simulink model "Model_RunAll"  (R2021b)
settings: Solver=FixedStepDiscrete  StartTime=0.0  StopTime=m.sys.tsim  FixedStep=p.sys.samp.tsim
values from neighbouring files (symbols this model uses):
  m = ConvertToDoublePrecision(m)    [Params.m]
  pp = Simulink.Parameter(p_single)    [Params.m]
settings Model: Creator=hamid.behjati  LastModifiedBy=behjati
settings DebuggingCC: AlgebraicLoopMsg=none  ParameterPrecisionLossMsg=none

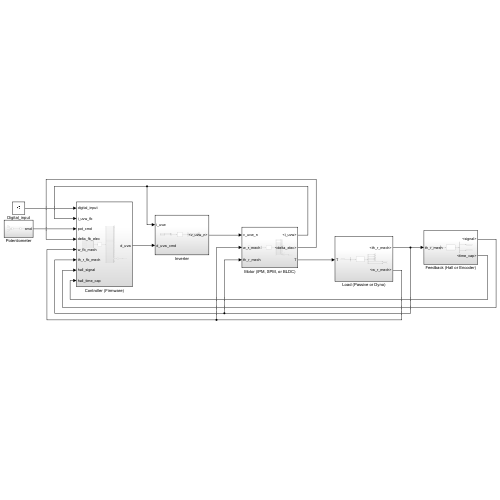
[thumbnail: Simulink's stored preview of the top-level diagram]
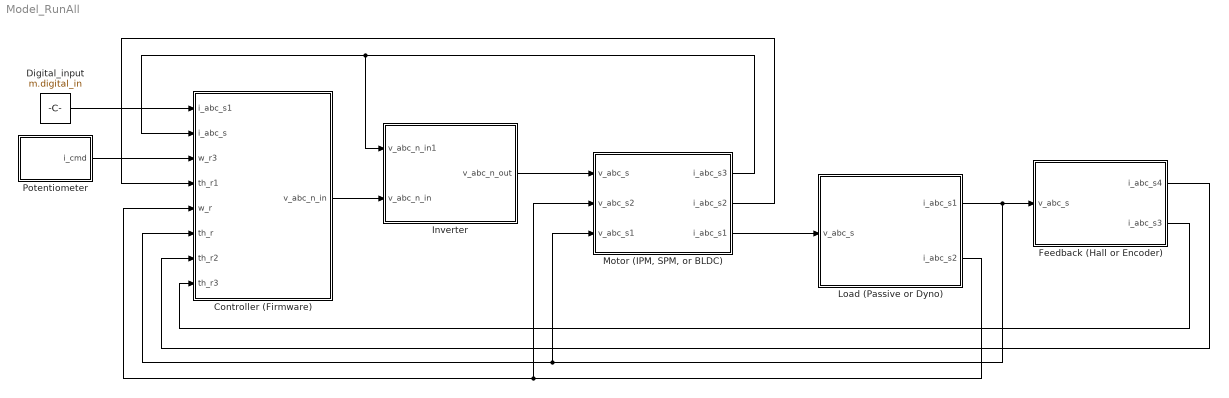
== system Model_RunAll ==
  Controller (Firmware) : Subsystem
  Digital_input : Constant  Value=m.digital_in
  Feedback (Hall or Encoder) : Subsystem
  Inverter : Subsystem
  Load (Passive or Dyno) : Subsystem
  "Motor (IPM, SPM, or BLDC)" : Subsystem
  Potentiometer : Subsystem
  wires:
  "Motor (IPM, SPM, or BLDC)"/3(i_abc_s1) -> Load (Passive or Dyno)/1(v_abc_s)
  "Motor (IPM, SPM, or BLDC)"/1(i_abc_s3) -> Controller (Firmware)/2(i_abc_s), Inverter/1(v_abc_n_in1)
  Potentiometer/1(i_cmd) -> Controller (Firmware)/3(w_r3)
  Controller (Firmware)/1(v_abc_n_in) -> Inverter/2(v_abc_n_in)
  Inverter/1(v_abc_n_out) -> "Motor (IPM, SPM, or BLDC)"/1(v_abc_s)
  Load (Passive or Dyno)/1(i_abc_s1) -> Feedback (Hall or Encoder)/1(v_abc_s), "Motor (IPM, SPM, or BLDC)"/3(v_abc_s1), Controller (Firmware)/6(th_r)
  "Motor (IPM, SPM, or BLDC)"/2(i_abc_s2) -> Controller (Firmware)/4(th_r1)
  Digital_input/1 -> Controller (Firmware)/1(i_abc_s1)
  Load (Passive or Dyno)/2(i_abc_s2) -> "Motor (IPM, SPM, or BLDC)"/2(v_abc_s2), Controller (Firmware)/5(w_r)
  Feedback (Hall or Encoder)/2(i_abc_s3) -> Controller (Firmware)/8(th_r3)
  Feedback (Hall or Encoder)/1(i_abc_s4) -> Controller (Firmware)/7(th_r2)

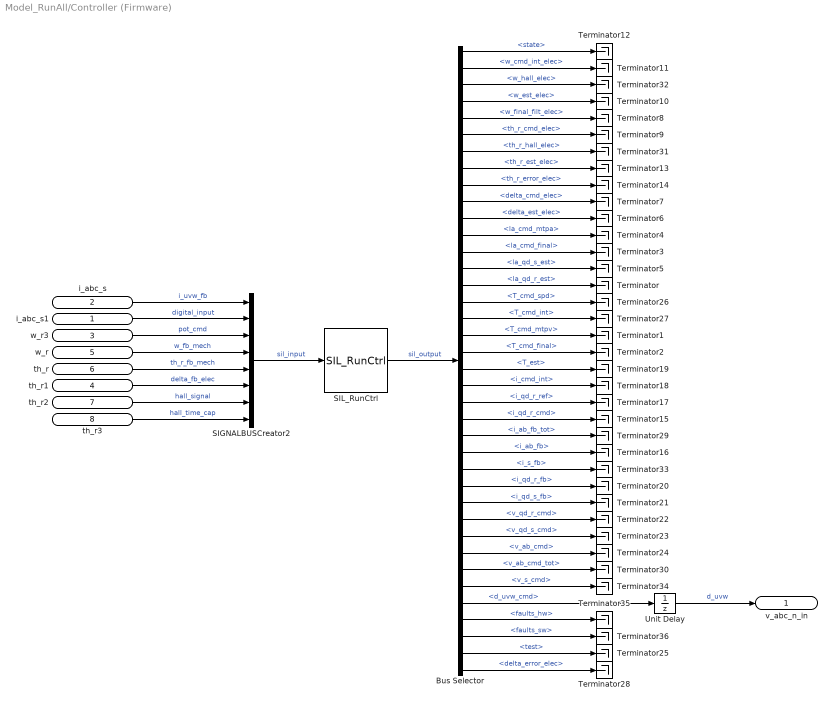
== system Model_RunAll/Controller (Firmware) ==
  i_abc_s1 : Inport
  i_abc_s : Inport  Port=2
  w_r3 : Inport  Port=3
  th_r1 : Inport  Port=4
  w_r : Inport  Port=5
  th_r : Inport  Port=6
  th_r2 : Inport  Port=7
  th_r3 : Inport  Port=8
  Bus Selector : BusSelector  OutputSignals=state,w_cmd_int_elec,w_hall_elec,w_est_elec,w_final_filt_elec,th_r_cmd_elec,th_r_hall_elec,th_r_est_elec,th_r_error_elec,delta_cmd_elec,delta_est_elec,la_cmd_mtpa,la_cmd_final,la_qd_s_est,la_qd_r_est,T_cmd_spd,T_cmd_int,T_cmd_mtpv,T_cmd_final,T_est,i_cmd_int,i_qd_r_ref,i_qd_r_cmd,i_ab_fb_tot,i_ab_fb,i_s_fb,i_qd_r_fb,i_qd_s_fb,v_qd_r_cmd,v_qd_s_cmd,v_ab_cmd,v_ab_cmd_tot,v_s_cmd,d_uvw_cmd,faults_hw,faults_sw,test,delta_error_elec
  SIGNALBUSCreator2 : BusCreator  Inputs=8  OutDataTypeStr=Bus: SIL_INPUT_CTRL_t
      settings: InheritFromInputs=off
  SIL_RunCtrl : S-Function  FunctionName=SIL_RunCtrl  Parameters=SParameter1  SFunctionDeploymentMode=off  EnableBusSupport=off  mask(Legacy Function){SFunctionSpec=void SIL_RunCtrl(SIL_INPUT_CTRL_t u1[1], SIL_OUTPUT_CTRL_t y1[1]), SParameter1=pp, ShowSpec=off}
      mask prompts: SParameter1 "P1:"; ShowSpec "Display function specification"
      mask help:
      | This block allows you to call the legacy functions specified by the following Legacy Code Tool definition:
      | def.SFunctionName = 'SIL_RunCtrl';
      | def.OutputFcnSpec = 'void SIL_RunCtrl(SIL_INPUT_CTRL_t u1[1], SIL_OUTPUT_CTRL_t y1[1])';
      | def.StartFcnSpec = 'void SIL_StartCtrl(PARAMS_t p1[1])';
      | def.TerminateFcnSpec = 'void SIL_TerminateCtrl()';
      | def.HeaderFiles = {'SILWrap.h'};
      | def.SourceFiles = {'Biquad.c', 'Controller.c', 'CtrlFilts.c', 'CtrlVars.c', 'FaultProtect.c', 'FluxWeaken.c', 'General.c', 'Observer.c', 'Params.c', 'PLL.c', 'ResonantFilt.c', 'SensorIface.c', 'SixPulseInj.c', 'SpeedCtrl.c', 'StateMachine.c', 'VoltCtrl.c', 'VoltMod.c', 'CInverter.cpp', 'CMechLoad.cpp', 'CMotor.cpp', 'AuxMethods.cpp', 'CPotentiometer.cpp', 'SILAuxFcns.cpp', 'SILWrap.cpp', 'DeltaCtrl.c', 'FluxCtrl.c', 'TrqCtrl.c'};
      | def.IncPaths = {'..\UnitTests\', '..\OperationalCode\'};
      | def.SrcPaths = {'..\UnitTests\', '..\OperationalCode\'};
      | def.SampleTime = 9.99999974737875e-06;
      mask Help: <p>This block was generated automatically by the Legacy Code Tool. For detailed help on this tool, call<a href="matlab:legacy_code('help')"> legacy_code('help')</a>.</p>
      mask Callback ShowSpec:
      | if strcmp(get_param(gcbh, 'ShowSpec'), 'on')
      |   set_param(gcbh, 'MaskDisplay', sprintf('fprintf(''%s'');', get_param(gcbh, 'SFunctionSpec')));
      | else
      |   set_param(gcbh, 'MaskDisplay', sprintf('fprintf(''%s'');', get_param(gcbh, 'FunctionName')));
      | end
      mask Display: fprintf('SIL_RunCtrl');
  Terminator{,1..36} (37 alike) : Terminator
  Unit Delay : UnitDelay  SampleTime=p.sys.samp.ts0  HasFrameUpgradeWarning=on
  v_abc_n_in : Outport
  wires:
  SIGNALBUSCreator2/1 -> SIL_RunCtrl/1  "sil_input"
  SIL_RunCtrl/1 -> Bus Selector/1  "sil_output"
  w_r/1 -> SIGNALBUSCreator2/4  "w_fb_mech"
  th_r/1 -> SIGNALBUSCreator2/5  "th_r_fb_mech"
  w_r3/1 -> SIGNALBUSCreator2/3  "pot_cmd"
  Bus Selector/1 -> Terminator12/1  "<state>"
  Bus Selector/2 -> Terminator11/1  "<w_cmd_int_elec>"
  Bus Selector/4 -> Terminator10/1  "<w_est_elec>"
  Bus Selector/5 -> Terminator8/1  "<w_final_filt_elec>"
  Bus Selector/6 -> Terminator9/1  "<th_r_cmd_elec>"
  Bus Selector/8 -> Terminator13/1  "<th_r_est_elec>"
  Bus Selector/9 -> Terminator14/1  "<th_r_error_elec>"
  Bus Selector/10 -> Terminator7/1  "<delta_cmd_elec>"
  Bus Selector/11 -> Terminator6/1  "<delta_est_elec>"
  Bus Selector/12 -> Terminator4/1  "<la_cmd_mtpa>"
  Bus Selector/13 -> Terminator3/1  "<la_cmd_final>"
  Bus Selector/15 -> Terminator/1  "<la_qd_r_est>"
  Bus Selector/18 -> Terminator1/1  "<T_cmd_mtpv>"
  Bus Selector/19 -> Terminator2/1  "<T_cmd_final>"
  Bus Selector/20 -> Terminator19/1  "<T_est>"
  Bus Selector/21 -> Terminator18/1  "<i_cmd_int>"
  Bus Selector/22 -> Terminator17/1  "<i_qd_r_ref>"
  Bus Selector/23 -> Terminator15/1  "<i_qd_r_cmd>"
  Bus Selector/37 -> Terminator25/1  "<test>"
  Bus Selector/17 -> Terminator27/1  "<T_cmd_int>"
  Bus Selector/16 -> Terminator26/1  "<T_cmd_spd>"
  Bus Selector/14 -> Terminator5/1  "<la_qd_s_est>"
  th_r1/1 -> SIGNALBUSCreator2/6  "delta_fb_elec"
  Bus Selector/38 -> Terminator28/1  "<delta_error_elec>"
  i_abc_s/1 -> SIGNALBUSCreator2/1  "i_uvw_fb"
  i_abc_s1/1 -> SIGNALBUSCreator2/2  "digital_input"
  Unit Delay/1 -> v_abc_n_in/1  "d_uvw"
  Bus Selector/34 -> Unit Delay/1  "<d_uvw_cmd>"
  th_r2/1 -> SIGNALBUSCreator2/7  "hall_signal"
  th_r3/1 -> SIGNALBUSCreator2/8  "hall_time_cap"
  Bus Selector/32 -> Terminator30/1  "<v_ab_cmd_tot>"
  Bus Selector/31 -> Terminator24/1  "<v_ab_cmd>"
  Bus Selector/30 -> Terminator23/1  "<v_qd_s_cmd>"
  Bus Selector/29 -> Terminator22/1  "<v_qd_r_cmd>"
  Bus Selector/28 -> Terminator21/1  "<i_qd_s_fb>"
  Bus Selector/27 -> Terminator20/1  "<i_qd_r_fb>"
  Bus Selector/25 -> Terminator16/1  "<i_ab_fb>"
  Bus Selector/24 -> Terminator29/1  "<i_ab_fb_tot>"
  Bus Selector/7 -> Terminator31/1  "<th_r_hall_elec>"
  Bus Selector/3 -> Terminator32/1  "<w_hall_elec>"
  Bus Selector/26 -> Terminator33/1  "<i_s_fb>"
  Bus Selector/33 -> Terminator34/1  "<v_s_cmd>"
  Bus Selector/35 -> Terminator35/1  "<faults_hw>"
  Bus Selector/36 -> Terminator36/1  "<faults_sw>"

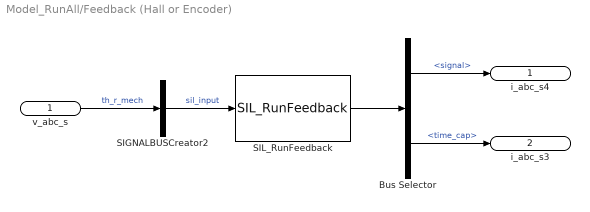
== system Model_RunAll/Feedback (Hall or Encoder) ==
  v_abc_s : Inport
  Bus Selector : BusSelector  OutputSignals=signal,time_cap
  SIGNALBUSCreator2 : BusCreator  Inputs=1  OutDataTypeStr=Bus: SIL_INPUT_FEEDBACK_t
      settings: InheritFromInputs=off
  SIL_RunFeedback : S-Function  FunctionName=SIL_RunFeedback  Parameters=SParameter1  SFunctionDeploymentMode=off  EnableBusSupport=off  mask(Legacy Function){SFunctionSpec=void SIL_RunFeedback(SIL_INPUT_FEEDBACK_t u1[1], SIL_OUTPUT_FEEDBACK_t y1[1]), SParameter1=pp, ShowSpec=off}
      mask prompts: SParameter1 "P1:"; ShowSpec "Display function specification"
      mask help:
      | This block allows you to call the legacy functions specified by the following Legacy Code Tool definition:
      | def.SFunctionName = 'SIL_RunFeedback';
      | def.OutputFcnSpec = 'void SIL_RunFeedback(SIL_INPUT_FEEDBACK_t u1[1], SIL_OUTPUT_FEEDBACK_t y1[1])';
      | def.StartFcnSpec = 'void SIL_StartFeedback(PARAMS_t p1[1])';
      | def.TerminateFcnSpec = 'void SIL_TerminateFeedback()';
      | def.HeaderFiles = {'SILWrapFeedback.h'};
      | def.SourceFiles = {'General.c', 'Params.c', 'ParamsDefault.c', 'CFeedback.cpp', 'CHallSensor.cpp', 'SILAuxFcns.cpp', 'AuxMethods.cpp', 'SILWrapFeedback.cpp'};
      | def.IncPaths = {'..\UnitTests\', '..\OperationalCode\'};
      | def.SrcPaths = {'..\UnitTests\', '..\OperationalCode\'};
      | def.SampleTime = 9.99999974737875e-06;
      mask Help: <p>This block was generated automatically by the Legacy Code Tool. For detailed help on this tool, call<a href="matlab:legacy_code('help')"> legacy_code('help')</a>.</p>
      mask Callback ShowSpec:
      | if strcmp(get_param(gcbh, 'ShowSpec'), 'on')
      |   set_param(gcbh, 'MaskDisplay', sprintf('fprintf(''%s'');', get_param(gcbh, 'SFunctionSpec')));
      | else
      |   set_param(gcbh, 'MaskDisplay', sprintf('fprintf(''%s'');', get_param(gcbh, 'FunctionName')));
      | end
      mask Display: fprintf('SIL_RunFeedback');
  i_abc_s4 : Outport
  i_abc_s3 : Outport  Port=2
  wires:
  SIL_RunFeedback/1 -> Bus Selector/1
  Bus Selector/1 -> i_abc_s4/1  "<signal>"
  Bus Selector/2 -> i_abc_s3/1  "<time_cap>"
  SIGNALBUSCreator2/1 -> SIL_RunFeedback/1  "sil_input"
  v_abc_s/1 -> SIGNALBUSCreator2/1  "th_r_mech"

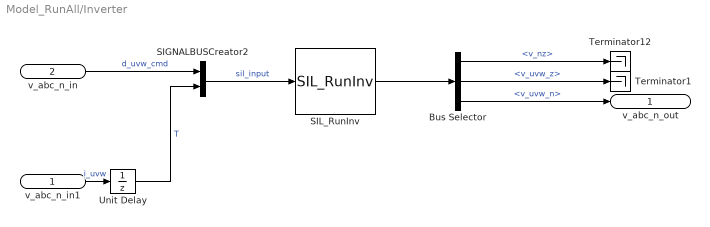
== system Model_RunAll/Inverter ==
  v_abc_n_in1 : Inport
  v_abc_n_in : Inport  Port=2
  Bus Selector : BusSelector  OutputSignals=v_nz,v_uvw_z,v_uvw_n
  SIGNALBUSCreator2 : BusCreator  Inputs=2  OutDataTypeStr=Bus: SIL_INPUT_INV_t
      settings: InheritFromInputs=off
  SIL_RunInv : S-Function  FunctionName=SIL_RunInv  Parameters=SParameter1  SFunctionDeploymentMode=off  EnableBusSupport=off  mask(Legacy Function){SFunctionSpec=void SIL_RunInv(SIL_INPUT_INV_t u1[1], SIL_OUTPUT_INV_t y1[1]), SParameter1=pp, ShowSpec=off}
      mask prompts: SParameter1 "P1:"; ShowSpec "Display function specification"
      mask help:
      | This block allows you to call the legacy functions specified by the following Legacy Code Tool definition:
      | def.SFunctionName = 'SIL_RunInv';
      | def.OutputFcnSpec = 'void SIL_RunInv(SIL_INPUT_INV_t u1[1], SIL_OUTPUT_INV_t y1[1])';
      | def.StartFcnSpec = 'void SIL_StartInv(PARAMS_t p1[1])';
      | def.TerminateFcnSpec = 'void SIL_TerminateInv()';
      | def.HeaderFiles = {'SILWrapInv.h'};
      | def.SourceFiles = {'General.c', 'Params.c', 'ParamsDefault.c', 'CInverter.cpp', 'SILAuxFcns.cpp', 'SILWrapInv.cpp'};
      | def.IncPaths = {'..\UnitTests\', '..\OperationalCode\'};
      | def.SrcPaths = {'..\UnitTests\', '..\OperationalCode\'};
      | def.SampleTime = 9.99999974737875e-06;
      mask Help: <p>This block was generated automatically by the Legacy Code Tool. For detailed help on this tool, call<a href="matlab:legacy_code('help')"> legacy_code('help')</a>.</p>
      mask Callback ShowSpec:
      | if strcmp(get_param(gcbh, 'ShowSpec'), 'on')
      |   set_param(gcbh, 'MaskDisplay', sprintf('fprintf(''%s'');', get_param(gcbh, 'SFunctionSpec')));
      | else
      |   set_param(gcbh, 'MaskDisplay', sprintf('fprintf(''%s'');', get_param(gcbh, 'FunctionName')));
      | end
      mask Display: fprintf('SIL_RunInv');
  Terminator1 : Terminator
  Terminator12 : Terminator
  Unit Delay : UnitDelay  SampleTime=p.sys.samp.tsim  HasFrameUpgradeWarning=on
  v_abc_n_out : Outport
  wires:
  SIL_RunInv/1 -> Bus Selector/1
  SIGNALBUSCreator2/1 -> SIL_RunInv/1  "sil_input"
  Bus Selector/2 -> Terminator1/1  "<v_uvw_z>"
  Bus Selector/1 -> Terminator12/1  "<v_nz>"
  Bus Selector/3 -> v_abc_n_out/1  "<v_uvw_n>"
  v_abc_n_in/1 -> SIGNALBUSCreator2/1  "d_uvw_cmd"
  v_abc_n_in1/1 -> Unit Delay/1  "i_uvw"
  Unit Delay/1 -> SIGNALBUSCreator2/2  "T"

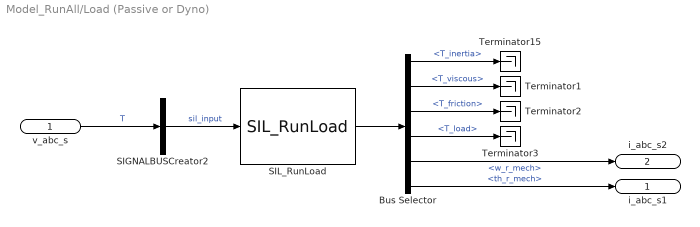
== system Model_RunAll/Load (Passive or Dyno) ==
  v_abc_s : Inport
  Bus Selector : BusSelector  OutputSignals=T_inertia,T_viscous,T_friction,T_load,w_r_mech,th_r_mech
  SIGNALBUSCreator2 : BusCreator  Inputs=1  OutDataTypeStr=Bus: SIL_INPUT_LOAD_t
      settings: InheritFromInputs=off
  SIL_RunLoad : S-Function  FunctionName=SIL_RunLoad  Parameters=SParameter1  SFunctionDeploymentMode=off  EnableBusSupport=off  mask(Legacy Function){SFunctionSpec=void SIL_RunLoad(SIL_INPUT_LOAD_t u1[1], SIL_OUTPUT_LOAD_t y1[1]), SParameter1=pp, ShowSpec=off}
      mask prompts: SParameter1 "P1:"; ShowSpec "Display function specification"
      mask help:
      | This block allows you to call the legacy functions specified by the following Legacy Code Tool definition:
      | def.SFunctionName = 'SIL_RunLoad';
      | def.OutputFcnSpec = 'void SIL_RunLoad(SIL_INPUT_LOAD_t u1[1], SIL_OUTPUT_LOAD_t y1[1])';
      | def.StartFcnSpec = 'void SIL_StartLoad(PARAMS_t p1[1])';
      | def.TerminateFcnSpec = 'void SIL_TerminateLoad()';
      | def.HeaderFiles = {'SILWrapLoad.h'};
      | def.SourceFiles = {'General.c', 'Params.c', 'ParamsDefault.c', 'CLoad.cpp', 'CMechLoad.cpp', 'CPotentiometer.cpp', 'CDyno.cpp', 'SILAuxFcns.cpp', 'AuxMethods.cpp', 'SILWrapLoad.cpp'};
      | def.IncPaths = {'..\UnitTests\', '..\OperationalCode\'};
      | def.SrcPaths = {'..\UnitTests\', '..\OperationalCode\'};
      | def.SampleTime = 9.99999974737875e-06;
      mask Help: <p>This block was generated automatically by the Legacy Code Tool. For detailed help on this tool, call<a href="matlab:legacy_code('help')"> legacy_code('help')</a>.</p>
      mask Callback ShowSpec:
      | if strcmp(get_param(gcbh, 'ShowSpec'), 'on')
      |   set_param(gcbh, 'MaskDisplay', sprintf('fprintf(''%s'');', get_param(gcbh, 'SFunctionSpec')));
      | else
      |   set_param(gcbh, 'MaskDisplay', sprintf('fprintf(''%s'');', get_param(gcbh, 'FunctionName')));
      | end
      mask Display: fprintf('SIL_RunLoad');
  Terminator{1..3,15} (4 alike) : Terminator
  i_abc_s1 : Outport
  i_abc_s2 : Outport  Port=2
  wires:
  SIL_RunLoad/1 -> Bus Selector/1
  Bus Selector/1 -> Terminator15/1  "<T_inertia>"
  Bus Selector/2 -> Terminator1/1  "<T_viscous>"
  Bus Selector/3 -> Terminator2/1  "<T_friction>"
  Bus Selector/4 -> Terminator3/1  "<T_load>"
  Bus Selector/5 -> i_abc_s2/1  "<w_r_mech>"
  SIGNALBUSCreator2/1 -> SIL_RunLoad/1  "sil_input"
  v_abc_s/1 -> SIGNALBUSCreator2/1  "T"
  Bus Selector/6 -> i_abc_s1/1  "<th_r_mech>"

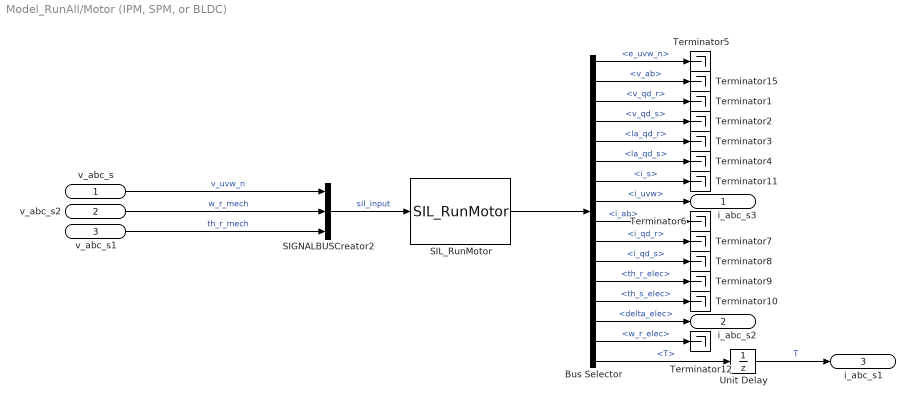
== system Model_RunAll/Motor (IPM, SPM, or BLDC) ==
  v_abc_s : Inport
  v_abc_s2 : Inport  Port=2
  v_abc_s1 : Inport  Port=3
  Bus Selector : BusSelector  OutputSignals=e_uvw_n,v_ab,v_qd_r,v_qd_s,la_qd_r,la_qd_s,i_s,i_uvw,i_ab,i_qd_r,i_qd_s,th_r_elec,th_s_elec,delta_elec,w_r_elec,T
  SIGNALBUSCreator2 : BusCreator  Inputs=3  OutDataTypeStr=Bus: SIL_INPUT_MOTOR_t
      settings: InheritFromInputs=off
  SIL_RunMotor : S-Function  FunctionName=SIL_RunMotor  Parameters=SParameter1  SFunctionDeploymentMode=off  EnableBusSupport=off  mask(Legacy Function){SFunctionSpec=void SIL_RunMotor(SIL_INPUT_MOTOR_t u1[1], SIL_OUTPUT_MOTOR_t y1[1]), SParameter1=pp, ShowSpec=off}
      mask prompts: SParameter1 "P1:"; ShowSpec "Display function specification"
      mask help:
      | This block allows you to call the legacy functions specified by the following Legacy Code Tool definition:
      | def.SFunctionName = 'SIL_RunMotor';
      | def.OutputFcnSpec = 'void SIL_RunMotor(SIL_INPUT_MOTOR_t u1[1], SIL_OUTPUT_MOTOR_t y1[1])';
      | def.StartFcnSpec = 'void SIL_StartMotor(PARAMS_t p1[1])';
      | def.TerminateFcnSpec = 'void SIL_TerminateMotor()';
      | def.HeaderFiles = {'SILWrapMotor.h'};
      | def.SourceFiles = {'General.c', 'Params.c', 'ParamsDefault.c', 'CMotor.cpp', 'CPMSM.cpp', 'CBLDC.cpp', 'SILAuxFcns.cpp', 'AuxMethods.cpp', 'SILWrapMotor.cpp'};
      | def.IncPaths = {'..\UnitTests\', '..\OperationalCode\'};
      | def.SrcPaths = {'..\UnitTests\', '..\OperationalCode\'};
      | def.SampleTime = 9.99999974737875e-06;
      mask Help: <p>This block was generated automatically by the Legacy Code Tool. For detailed help on this tool, call<a href="matlab:legacy_code('help')"> legacy_code('help')</a>.</p>
      mask Callback ShowSpec:
      | if strcmp(get_param(gcbh, 'ShowSpec'), 'on')
      |   set_param(gcbh, 'MaskDisplay', sprintf('fprintf(''%s'');', get_param(gcbh, 'SFunctionSpec')));
      | else
      |   set_param(gcbh, 'MaskDisplay', sprintf('fprintf(''%s'');', get_param(gcbh, 'FunctionName')));
      | end
      mask Display: fprintf('SIL_RunMotor');
  Terminator{1..12,15} (13 alike) : Terminator
  Unit Delay : UnitDelay  SampleTime=p.sys.samp.tsim  HasFrameUpgradeWarning=on
  i_abc_s3 : Outport
  i_abc_s2 : Outport  Port=2
  i_abc_s1 : Outport  Port=3
  wires:
  SIGNALBUSCreator2/1 -> SIL_RunMotor/1  "sil_input"
  SIL_RunMotor/1 -> Bus Selector/1
  Bus Selector/2 -> Terminator15/1  "<v_ab>"
  Bus Selector/3 -> Terminator1/1  "<v_qd_r>"
  Bus Selector/4 -> Terminator2/1  "<v_qd_s>"
  Bus Selector/5 -> Terminator3/1  "<la_qd_r>"
  Bus Selector/6 -> Terminator4/1  "<la_qd_s>"
  Bus Selector/8 -> i_abc_s3/1  "<i_uvw>"
  Bus Selector/9 -> Terminator6/1  "<i_ab>"
  Bus Selector/10 -> Terminator7/1  "<i_qd_r>"
  Bus Selector/11 -> Terminator8/1  "<i_qd_s>"
  Bus Selector/12 -> Terminator9/1  "<th_r_elec>"
  Bus Selector/13 -> Terminator10/1  "<th_s_elec>"
  Bus Selector/14 -> i_abc_s2/1  "<delta_elec>"
  Bus Selector/15 -> Terminator12/1  "<w_r_elec>"
  v_abc_s/1 -> SIGNALBUSCreator2/1  "v_uvw_n"
  v_abc_s2/1 -> SIGNALBUSCreator2/2  "w_r_mech"
  v_abc_s1/1 -> SIGNALBUSCreator2/3  "th_r_mech"
  Bus Selector/16 -> Unit Delay/1  "<T>"
  Unit Delay/1 -> i_abc_s1/1  "T"
  Bus Selector/1 -> Terminator5/1  "<e_uvw_n>"
  Bus Selector/7 -> Terminator11/1  "<i_s>"

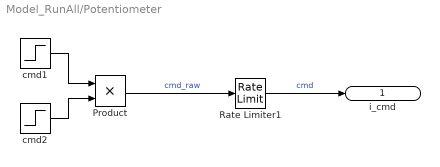
== system Model_RunAll/Potentiometer ==
  Product : Product
  Rate Limiter1 : RateLimiter  RisingSlewLimit=m.pot.slope_lim  FallingSlewLimit=-m.pot.slope_lim  SampleTimeMode=inherited
  cmd1 : Step  Time=m.pot.t_start  Before=m.pot.init/sqrt(m.pot.final)  After=sqrt(m.pot.final)  SampleTime=0
  cmd2 : Step  Time=m.pot.t_stop  Before=sqrt(m.pot.final)  After=m.pot.init/sqrt(m.pot.final)  SampleTime=0
  i_cmd : Outport
  wires:
  cmd1/1 -> Product/1
  cmd2/1 -> Product/2
  Rate Limiter1/1 -> i_cmd/1  "cmd"
  Product/1 -> Rate Limiter1/1  "cmd_raw"
